simulink model "VCU_CS75_12_27_test"  (R2014a)
settings: Solver=FixedStepDiscrete  StartTime=0.0  StopTime=25  FixedStep=0.0005  RelTol=1e-3
undefined symbols (not defined in the file): D1, D2, D3, ecucoder_acal, ErrorSumMax1, ErrorSumMax2, ErrorSumMax3, I1, I2, I3, I_SW01_L, LaterlAngleCommand, LDW, P1, P2, P3, RemoteAcclPosition
libraries: simulink x913, ec5744lib x39
(part 11 of 30)

== system VCU_CS75_12_27_test/长安CS75底盘程序，20ms一次/Output/Subsystem/TransmitMessages10/LAS_29D ==
  LAS_LASWarningModeSelectionSts_in : Inport
  LAS_SLASwitchStatus_in : Inport  Port=2
  LAS_HMAEnableStatus_in : Inport  Port=3
  LAS_LASModeSelectionStatus_in : Inport  Port=4
  LAS_LdwSensitivityStatus_in : Inport  Port=5
  LAS_OverspeedSoundWarningEnSt_in : Inport  Port=6
  LAS_FatigueDectionEnableStatus_in : Inport  Port=7
  LAS_LDWShakeLevStatus_in : Inport  Port=8
  LAS_HostLaneLeftStatus_in : Inport  Port=9
  LAS_VoiceWarning_in : Inport  Port=10
  LAS_HostLaneRightStatus_in : Inport  Port=11
  LAS_OverspeedWarningEnableStatus_in : Inport  Port=12
  LAS_OverspeedSoundWarning_in : Inport  Port=13
  LAS_LLaneMarkerType_in : Inport  Port=14
  LAS_OverspeedVisualWarning_in : Inport  Port=15
  LAS_RLaneMarkerType_in : Inport  Port=16
  LAS_OverspeedWarningOffset_in : Inport  Port=17
  RollingConter_in : Inport  Port=18
  LAS_IACCEnableStatus_in : Inport  Port=19
  CRC_in : Inport  Port=20
  CRC : Subsystem
  Conv{1..8} (8 alike) : DataTypeConversion
  LAS_29D_DLC : Constant  Value=8  OutDataTypeStr=uint8
  LAS_29D_DLC_Out : Terminator
  LAS_29D_ID : Constant  Value=669  OutDataTypeStr=single
  LAS_29D_ID_Out : Terminator
  LAS_29D_mux : Mux  Inputs=8
  LAS_FatigueDectionEnableStatus : Subsystem
  LAS_HMAEnableStatus : Subsystem
  LAS_HostLaneLeftStatus : Subsystem
  LAS_HostLaneRightStatus : Subsystem
  LAS_IACCEnableStatus : Subsystem
  LAS_LASModeSelectionStatus : Subsystem
  LAS_LASWarningModeSelectionSts : Subsystem
  LAS_LDWShakeLevStatus : Subsystem
  LAS_LLaneMarkerType : Subsystem
  LAS_LdwSensitivityStatus : Subsystem
  LAS_OverspeedSoundWarning : Subsystem
  LAS_OverspeedSoundWarningEnSt : Subsystem
  LAS_OverspeedVisualWarning : Subsystem
  LAS_OverspeedWarningEnableStatus : Subsystem
  LAS_OverspeedWarningOffset : Subsystem
  LAS_RLaneMarkerType : Subsystem
  LAS_SLASwitchStatus : Subsystem
  LAS_VoiceWarning : Subsystem
  RollingConter : Subsystem
  or{1..8} (8 alike) : simulink/Logic and Bit Operations/Bitwise Operator  logicop=OR  UseBitMask=off  NumInputPorts=20  BitMask=bin2dec('11011001')  BitMaskRealWorld=Stored Integer
  output : Outport
  wires:
  LAS_29D_mux/1 -> output/1
  LAS_LASWarningModeSelectionSts/1(output1) -> or1/1
  LAS_LASWarningModeSelectionSts/2(output2) -> or2/1
  LAS_LASWarningModeSelectionSts/3(output3) -> or3/1
  LAS_LASWarningModeSelectionSts/4(output4) -> or4/1
  LAS_LASWarningModeSelectionSts/5(output5) -> or5/1
  LAS_LASWarningModeSelectionSts/6(output6) -> or6/1
  LAS_LASWarningModeSelectionSts/7(output7) -> or7/1
  LAS_LASWarningModeSelectionSts/8(output8) -> or8/1
  LAS_SLASwitchStatus/1(output1) -> or1/2
  LAS_SLASwitchStatus/2(output2) -> or2/2
  LAS_SLASwitchStatus/3(output3) -> or3/2
  LAS_SLASwitchStatus/4(output4) -> or4/2
  LAS_SLASwitchStatus/5(output5) -> or5/2
  LAS_SLASwitchStatus/6(output6) -> or6/2
  LAS_SLASwitchStatus/7(output7) -> or7/2
  LAS_SLASwitchStatus/8(output8) -> or8/2
  LAS_HMAEnableStatus/1(output1) -> or1/3
  LAS_HMAEnableStatus/2(output2) -> or2/3
  LAS_HMAEnableStatus/3(output3) -> or3/3
  LAS_HMAEnableStatus/4(output4) -> or4/3
  LAS_HMAEnableStatus/5(output5) -> or5/3
  LAS_HMAEnableStatus/6(output6) -> or6/3
  LAS_HMAEnableStatus/7(output7) -> or7/3
  LAS_HMAEnableStatus/8(output8) -> or8/3
  LAS_LASModeSelectionStatus/1(output1) -> or1/4
  LAS_LASModeSelectionStatus/2(output2) -> or2/4
  LAS_LASModeSelectionStatus/3(output3) -> or3/4
  LAS_LASModeSelectionStatus/4(output4) -> or4/4
  LAS_LASModeSelectionStatus/5(output5) -> or5/4
  LAS_LASModeSelectionStatus/6(output6) -> or6/4
  LAS_LASModeSelectionStatus/7(output7) -> or7/4
  LAS_LASModeSelectionStatus/8(output8) -> or8/4
  LAS_LdwSensitivityStatus/1(output1) -> or1/5
  LAS_LdwSensitivityStatus/2(output2) -> or2/5
  LAS_LdwSensitivityStatus/3(output3) -> or3/5
  LAS_LdwSensitivityStatus/4(output4) -> or4/5
  LAS_LdwSensitivityStatus/5(output5) -> or5/5
  LAS_LdwSensitivityStatus/6(output6) -> or6/5
  LAS_LdwSensitivityStatus/7(output7) -> or7/5
  LAS_LdwSensitivityStatus/8(output8) -> or8/5
  LAS_OverspeedSoundWarningEnSt/1(output1) -> or1/6
  LAS_OverspeedSoundWarningEnSt/2(output2) -> or2/6
  LAS_OverspeedSoundWarningEnSt/3(output3) -> or3/6
  LAS_OverspeedSoundWarningEnSt/4(output4) -> or4/6
  LAS_OverspeedSoundWarningEnSt/5(output5) -> or5/6
  LAS_OverspeedSoundWarningEnSt/6(output6) -> or6/6
  LAS_OverspeedSoundWarningEnSt/7(output7) -> or7/6
  LAS_OverspeedSoundWarningEnSt/8(output8) -> or8/6
  LAS_FatigueDectionEnableStatus/1(output1) -> or1/7
  LAS_FatigueDectionEnableStatus/2(output2) -> or2/7
  LAS_FatigueDectionEnableStatus/3(output3) -> or3/7
  LAS_FatigueDectionEnableStatus/4(output4) -> or4/7
  LAS_FatigueDectionEnableStatus/5(output5) -> or5/7
  LAS_FatigueDectionEnableStatus/6(output6) -> or6/7
  LAS_FatigueDectionEnableStatus/7(output7) -> or7/7
  LAS_FatigueDectionEnableStatus/8(output8) -> or8/7
  LAS_LDWShakeLevStatus/1(output1) -> or1/8
  LAS_LDWShakeLevStatus/2(output2) -> or2/8
  LAS_LDWShakeLevStatus/3(output3) -> or3/8
  LAS_LDWShakeLevStatus/4(output4) -> or4/8
  LAS_LDWShakeLevStatus/5(output5) -> or5/8
  LAS_LDWShakeLevStatus/6(output6) -> or6/8
  LAS_LDWShakeLevStatus/7(output7) -> or7/8
  LAS_LDWShakeLevStatus/8(output8) -> or8/8
  LAS_HostLaneLeftStatus/1(output1) -> or1/9
  LAS_HostLaneLeftStatus/2(output2) -> or2/9
  LAS_HostLaneLeftStatus/3(output3) -> or3/9
  LAS_HostLaneLeftStatus/4(output4) -> or4/9
  LAS_HostLaneLeftStatus/5(output5) -> or5/9
  LAS_HostLaneLeftStatus/6(output6) -> or6/9
  LAS_HostLaneLeftStatus/7(output7) -> or7/9
  LAS_HostLaneLeftStatus/8(output8) -> or8/9
  LAS_VoiceWarning/1(output1) -> or1/10
  LAS_VoiceWarning/2(output2) -> or2/10
  LAS_VoiceWarning/3(output3) -> or3/10
  LAS_VoiceWarning/4(output4) -> or4/10
  LAS_VoiceWarning/5(output5) -> or5/10
  LAS_VoiceWarning/6(output6) -> or6/10
  LAS_VoiceWarning/7(output7) -> or7/10
  LAS_VoiceWarning/8(output8) -> or8/10
  LAS_HostLaneRightStatus/1(output1) -> or1/11
  LAS_HostLaneRightStatus/2(output2) -> or2/11
  LAS_HostLaneRightStatus/3(output3) -> or3/11
  LAS_HostLaneRightStatus/4(output4) -> or4/11
  LAS_HostLaneRightStatus/5(output5) -> or5/11
  LAS_HostLaneRightStatus/6(output6) -> or6/11
  LAS_HostLaneRightStatus/7(output7) -> or7/11
  LAS_HostLaneRightStatus/8(output8) -> or8/11
  LAS_OverspeedWarningEnableStatus/1(output1) -> or1/12
  LAS_OverspeedWarningEnableStatus/2(output2) -> or2/12
  LAS_OverspeedWarningEnableStatus/3(output3) -> or3/12
  LAS_OverspeedWarningEnableStatus/4(output4) -> or4/12
  LAS_OverspeedWarningEnableStatus/5(output5) -> or5/12
  LAS_OverspeedWarningEnableStatus/6(output6) -> or6/12
  LAS_OverspeedWarningEnableStatus/7(output7) -> or7/12
  LAS_OverspeedWarningEnableStatus/8(output8) -> or8/12
  LAS_OverspeedSoundWarning/1(output1) -> or1/13
  LAS_OverspeedSoundWarning/2(output2) -> or2/13
  LAS_OverspeedSoundWarning/3(output3) -> or3/13
  LAS_OverspeedSoundWarning/4(output4) -> or4/13
  LAS_OverspeedSoundWarning/5(output5) -> or5/13
  LAS_OverspeedSoundWarning/6(output6) -> or6/13
  LAS_OverspeedSoundWarning/7(output7) -> or7/13
  LAS_OverspeedSoundWarning/8(output8) -> or8/13
  LAS_LLaneMarkerType/1(output1) -> or1/14
  LAS_LLaneMarkerType/2(output2) -> or2/14
  LAS_LLaneMarkerType/3(output3) -> or3/14
  LAS_LLaneMarkerType/4(output4) -> or4/14
  LAS_LLaneMarkerType/5(output5) -> or5/14
  LAS_LLaneMarkerType/6(output6) -> or6/14
  LAS_LLaneMarkerType/7(output7) -> or7/14
  LAS_LLaneMarkerType/8(output8) -> or8/14
  LAS_OverspeedVisualWarning/1(output1) -> or1/15
  LAS_OverspeedVisualWarning/2(output2) -> or2/15
  LAS_OverspeedVisualWarning/3(output3) -> or3/15
  LAS_OverspeedVisualWarning/4(output4) -> or4/15
  LAS_OverspeedVisualWarning/5(output5) -> or5/15
  LAS_OverspeedVisualWarning/6(output6) -> or6/15
  LAS_OverspeedVisualWarning/7(output7) -> or7/15
  LAS_OverspeedVisualWarning/8(output8) -> or8/15
  LAS_RLaneMarkerType/1(output1) -> or1/16
  LAS_RLaneMarkerType/2(output2) -> or2/16
  LAS_RLaneMarkerType/3(output3) -> or3/16
  LAS_RLaneMarkerType/4(output4) -> or4/16
  LAS_RLaneMarkerType/5(output5) -> or5/16
  LAS_RLaneMarkerType/6(output6) -> or6/16
  LAS_RLaneMarkerType/7(output7) -> or7/16
  LAS_RLaneMarkerType/8(output8) -> or8/16
  LAS_OverspeedWarningOffset/1(output1) -> or1/17
  LAS_OverspeedWarningOffset/2(output2) -> or2/17
  LAS_OverspeedWarningOffset/3(output3) -> or3/17
  LAS_OverspeedWarningOffset/4(output4) -> or4/17
  LAS_OverspeedWarningOffset/5(output5) -> or5/17
  LAS_OverspeedWarningOffset/6(output6) -> or6/17
  LAS_OverspeedWarningOffset/7(output7) -> or7/17
  LAS_OverspeedWarningOffset/8(output8) -> or8/17
  RollingConter/1(output1) -> or1/18
  RollingConter/2(output2) -> or2/18
  RollingConter/3(output3) -> or3/18
  RollingConter/4(output4) -> or4/18
  RollingConter/5(output5) -> or5/18
  RollingConter/6(output6) -> or6/18
  RollingConter/7(output7) -> or7/18
  RollingConter/8(output8) -> or8/18
  LAS_IACCEnableStatus/1(output1) -> or1/19
  LAS_IACCEnableStatus/2(output2) -> or2/19
  LAS_IACCEnableStatus/3(output3) -> or3/19
  LAS_IACCEnableStatus/4(output4) -> or4/19
  LAS_IACCEnableStatus/5(output5) -> or5/19
  LAS_IACCEnableStatus/6(output6) -> or6/19
  LAS_IACCEnableStatus/7(output7) -> or7/19
  LAS_IACCEnableStatus/8(output8) -> or8/19
  CRC/1(output1) -> or1/20
  CRC/2(output2) -> or2/20
  CRC/3(output3) -> or3/20
  CRC/4(output4) -> or4/20
  CRC/5(output5) -> or5/20
  CRC/6(output6) -> or6/20
  CRC/7(output7) -> or7/20
  CRC/8(output8) -> or8/20
  or1/1 -> Conv1/1
  Conv1/1 -> LAS_29D_mux/1
  or2/1 -> Conv2/1
  Conv2/1 -> LAS_29D_mux/2
  or3/1 -> Conv3/1
  Conv3/1 -> LAS_29D_mux/3
  or4/1 -> Conv4/1
  Conv4/1 -> LAS_29D_mux/4
  or5/1 -> Conv5/1
  Conv5/1 -> LAS_29D_mux/5
  or6/1 -> Conv6/1
  Conv6/1 -> LAS_29D_mux/6
  or7/1 -> Conv7/1
  Conv7/1 -> LAS_29D_mux/7
  or8/1 -> Conv8/1
  Conv8/1 -> LAS_29D_mux/8
  LAS_29D_ID/1 -> LAS_29D_ID_Out/1
  LAS_29D_DLC/1 -> LAS_29D_DLC_Out/1
  LAS_LASWarningModeSelectionSts_in/1 -> LAS_LASWarningModeSelectionSts/1(LAS_LASWarningModeSelectionSts)
  LAS_SLASwitchStatus_in/1 -> LAS_SLASwitchStatus/1(LAS_SLASwitchStatus)
  LAS_HMAEnableStatus_in/1 -> LAS_HMAEnableStatus/1(LAS_HMAEnableStatus)
  LAS_LASModeSelectionStatus_in/1 -> LAS_LASModeSelectionStatus/1(LAS_LASModeSelectionStatus)
  LAS_LdwSensitivityStatus_in/1 -> LAS_LdwSensitivityStatus/1(LAS_LdwSensitivityStatus)
  LAS_OverspeedSoundWarningEnSt_in/1 -> LAS_OverspeedSoundWarningEnSt/1(LAS_OverspeedSoundWarningEnSt)
  LAS_FatigueDectionEnableStatus_in/1 -> LAS_FatigueDectionEnableStatus/1(LAS_FatigueDectionEnableStatus)
  LAS_LDWShakeLevStatus_in/1 -> LAS_LDWShakeLevStatus/1(LAS_LDWShakeLevStatus)
  LAS_HostLaneLeftStatus_in/1 -> LAS_HostLaneLeftStatus/1(LAS_HostLaneLeftStatus)
  LAS_VoiceWarning_in/1 -> LAS_VoiceWarning/1(LAS_VoiceWarning)
  LAS_HostLaneRightStatus_in/1 -> LAS_HostLaneRightStatus/1(LAS_HostLaneRightStatus)
  LAS_OverspeedWarningEnableStatus_in/1 -> LAS_OverspeedWarningEnableStatus/1(LAS_OverspeedWarningEnableStatus)
  LAS_OverspeedSoundWarning_in/1 -> LAS_OverspeedSoundWarning/1(LAS_OverspeedSoundWarning)
  LAS_LLaneMarkerType_in/1 -> LAS_LLaneMarkerType/1(LAS_LLaneMarkerType)
  LAS_OverspeedVisualWarning_in/1 -> LAS_OverspeedVisualWarning/1(LAS_OverspeedVisualWarning)
  LAS_RLaneMarkerType_in/1 -> LAS_RLaneMarkerType/1(LAS_RLaneMarkerType)
  LAS_OverspeedWarningOffset_in/1 -> LAS_OverspeedWarningOffset/1(LAS_OverspeedWarningOffset)
  RollingConter_in/1 -> RollingConter/1(RollingConter)
  LAS_IACCEnableStatus_in/1 -> LAS_IACCEnableStatus/1(LAS_IACCEnableStatus)
  CRC_in/1 -> CRC/1(CRC)

== system VCU_CS75_12_27_test/长安CS75底盘程序，20ms一次/Output/Subsystem/TransmitMessages11/GW_LCDAL_2EA ==
  LCDAL_SystemStatus_in : Inport
  LCDAL_BSDLCAEnableStatus_in : Inport  Port=2
  LCDAL_BSDLCAAlert_in : Inport  Port=3
  LCDAL_BSDLCAStatus_in : Inport  Port=4
  LCDAL_CTAEnableStatus_in : Inport  Port=5
  LCDAL_CTAAlert_in : Inport  Port=6
  LCDAL_CTAStatus_in : Inport  Port=7
  LCDAL_RCWEnableStatus_in : Inport  Port=8
  LCDAL_RCWAlert_in : Inport  Port=9
  LCDAL_RCWStatus_in : Inport  Port=10
  LCDAL_RCWSoundEnableStatus_in : Inport  Port=11
  LCDAL_SEAEnableStatus_in : Inport  Port=12
  LCDAL_SEAAlert_in : Inport  Port=13
  LCDAL_SEAStatus_in : Inport  Port=14
  LCDAL_AudioWarningEnableStatus_in : Inport  Port=15
  LCDAL_LockCtrlEnableStatus_in : Inport  Port=16
  LCDAL_LCATTCSettingStatus_in : Inport  Port=17
  Conv{1..8} (8 alike) : DataTypeConversion
  GW_LCDAL_2EA_DLC : Constant  Value=8  OutDataTypeStr=uint8
  GW_LCDAL_2EA_DLC_Out : Terminator
  GW_LCDAL_2EA_ID : Constant  Value=746  OutDataTypeStr=single
  GW_LCDAL_2EA_ID_Out : Terminator
  GW_LCDAL_2EA_mux : Mux  Inputs=8
  LCDAL_AudioWarningEnableStatus : Subsystem
  LCDAL_BSDLCAAlert : Subsystem
  LCDAL_BSDLCAEnableStatus : Subsystem
  LCDAL_BSDLCAStatus : Subsystem
  LCDAL_CTAAlert : Subsystem
  LCDAL_CTAEnableStatus : Subsystem
  LCDAL_CTAStatus : Subsystem
  LCDAL_LCATTCSettingStatus : Subsystem
  LCDAL_LockCtrlEnableStatus : Subsystem
  LCDAL_RCWAlert : Subsystem
  LCDAL_RCWEnableStatus : Subsystem
  LCDAL_RCWSoundEnableStatus : Subsystem
  LCDAL_RCWStatus : Subsystem
  LCDAL_SEAAlert : Subsystem
  LCDAL_SEAEnableStatus : Subsystem
  LCDAL_SEAStatus : Subsystem
  LCDAL_SystemStatus : Subsystem
  or{1..8} (8 alike) : simulink/Logic and Bit Operations/Bitwise Operator  logicop=OR  UseBitMask=off  NumInputPorts=17  BitMask=bin2dec('11011001')  BitMaskRealWorld=Stored Integer
  output : Outport
  wires:
  LCDAL_LCATTCSettingStatus_in/1 -> LCDAL_LCATTCSettingStatus/1(LCDAL_LCATTCSettingStatus)
  LCDAL_LockCtrlEnableStatus_in/1 -> LCDAL_LockCtrlEnableStatus/1(LCDAL_LockCtrlEnableStatus)
  LCDAL_AudioWarningEnableStatus_in/1 -> LCDAL_AudioWarningEnableStatus/1(LCDAL_AudioWarningEnableStatus)
  LCDAL_SEAStatus_in/1 -> LCDAL_SEAStatus/1(LCDAL_SEAStatus)
  LCDAL_SEAAlert_in/1 -> LCDAL_SEAAlert/1(LCDAL_SEAAlert)
  LCDAL_SEAEnableStatus_in/1 -> LCDAL_SEAEnableStatus/1(LCDAL_SEAEnableStatus)
  LCDAL_RCWSoundEnableStatus_in/1 -> LCDAL_RCWSoundEnableStatus/1(LCDAL_RCWSoundEnableStatus)
  LCDAL_RCWStatus_in/1 -> LCDAL_RCWStatus/1(LCDAL_RCWStatus)
  LCDAL_RCWAlert_in/1 -> LCDAL_RCWAlert/1(LCDAL_RCWAlert)
  LCDAL_RCWEnableStatus_in/1 -> LCDAL_RCWEnableStatus/1(LCDAL_RCWEnableStatus)
  LCDAL_CTAStatus_in/1 -> LCDAL_CTAStatus/1(LCDAL_CTAStatus)
  LCDAL_CTAAlert_in/1 -> LCDAL_CTAAlert/1(LCDAL_CTAAlert)
  LCDAL_CTAEnableStatus_in/1 -> LCDAL_CTAEnableStatus/1(LCDAL_CTAEnableStatus)
  LCDAL_BSDLCAStatus_in/1 -> LCDAL_BSDLCAStatus/1(LCDAL_BSDLCAStatus)
  LCDAL_BSDLCAAlert_in/1 -> LCDAL_BSDLCAAlert/1(LCDAL_BSDLCAAlert)
  LCDAL_BSDLCAEnableStatus_in/1 -> LCDAL_BSDLCAEnableStatus/1(LCDAL_BSDLCAEnableStatus)
  LCDAL_SystemStatus_in/1 -> LCDAL_SystemStatus/1(LCDAL_SystemStatus)
  GW_LCDAL_2EA_DLC/1 -> GW_LCDAL_2EA_DLC_Out/1
  GW_LCDAL_2EA_ID/1 -> GW_LCDAL_2EA_ID_Out/1
  Conv8/1 -> GW_LCDAL_2EA_mux/8
  or8/1 -> Conv8/1
  Conv7/1 -> GW_LCDAL_2EA_mux/7
  or7/1 -> Conv7/1
  Conv6/1 -> GW_LCDAL_2EA_mux/6
  or6/1 -> Conv6/1
  Conv5/1 -> GW_LCDAL_2EA_mux/5
  or5/1 -> Conv5/1
  Conv4/1 -> GW_LCDAL_2EA_mux/4
  or4/1 -> Conv4/1
  Conv3/1 -> GW_LCDAL_2EA_mux/3
  or3/1 -> Conv3/1
  Conv2/1 -> GW_LCDAL_2EA_mux/2
  or2/1 -> Conv2/1
  Conv1/1 -> GW_LCDAL_2EA_mux/1
  or1/1 -> Conv1/1
  LCDAL_LCATTCSettingStatus/8(output8) -> or8/17
  LCDAL_LCATTCSettingStatus/7(output7) -> or7/17
  LCDAL_LCATTCSettingStatus/6(output6) -> or6/17
  LCDAL_LCATTCSettingStatus/5(output5) -> or5/17
  LCDAL_LCATTCSettingStatus/4(output4) -> or4/17
  LCDAL_LCATTCSettingStatus/3(output3) -> or3/17
  LCDAL_LCATTCSettingStatus/2(output2) -> or2/17
  LCDAL_LCATTCSettingStatus/1(output1) -> or1/17
  LCDAL_LockCtrlEnableStatus/8(output8) -> or8/16
  LCDAL_LockCtrlEnableStatus/7(output7) -> or7/16
  LCDAL_LockCtrlEnableStatus/6(output6) -> or6/16
  LCDAL_LockCtrlEnableStatus/5(output5) -> or5/16
  LCDAL_LockCtrlEnableStatus/4(output4) -> or4/16
  LCDAL_LockCtrlEnableStatus/3(output3) -> or3/16
  LCDAL_LockCtrlEnableStatus/2(output2) -> or2/16
  LCDAL_LockCtrlEnableStatus/1(output1) -> or1/16
  LCDAL_AudioWarningEnableStatus/8(output8) -> or8/15
  LCDAL_AudioWarningEnableStatus/7(output7) -> or7/15
  LCDAL_AudioWarningEnableStatus/6(output6) -> or6/15
  LCDAL_AudioWarningEnableStatus/5(output5) -> or5/15
  LCDAL_AudioWarningEnableStatus/4(output4) -> or4/15
  LCDAL_AudioWarningEnableStatus/3(output3) -> or3/15
  LCDAL_AudioWarningEnableStatus/2(output2) -> or2/15
  LCDAL_AudioWarningEnableStatus/1(output1) -> or1/15
  LCDAL_SEAStatus/8(output8) -> or8/14
  LCDAL_SEAStatus/7(output7) -> or7/14
  LCDAL_SEAStatus/6(output6) -> or6/14
  LCDAL_SEAStatus/5(output5) -> or5/14
  LCDAL_SEAStatus/4(output4) -> or4/14
  LCDAL_SEAStatus/3(output3) -> or3/14
  LCDAL_SEAStatus/2(output2) -> or2/14
  LCDAL_SEAStatus/1(output1) -> or1/14
  LCDAL_SEAAlert/8(output8) -> or8/13
  LCDAL_SEAAlert/7(output7) -> or7/13
  LCDAL_SEAAlert/6(output6) -> or6/13
  LCDAL_SEAAlert/5(output5) -> or5/13
  LCDAL_SEAAlert/4(output4) -> or4/13
  LCDAL_SEAAlert/3(output3) -> or3/13
  LCDAL_SEAAlert/2(output2) -> or2/13
  LCDAL_SEAAlert/1(output1) -> or1/13
  LCDAL_SEAEnableStatus/8(output8) -> or8/12
  LCDAL_SEAEnableStatus/7(output7) -> or7/12
  LCDAL_SEAEnableStatus/6(output6) -> or6/12
  LCDAL_SEAEnableStatus/5(output5) -> or5/12
  LCDAL_SEAEnableStatus/4(output4) -> or4/12
  LCDAL_SEAEnableStatus/3(output3) -> or3/12
  LCDAL_SEAEnableStatus/2(output2) -> or2/12
  LCDAL_SEAEnableStatus/1(output1) -> or1/12
  LCDAL_RCWSoundEnableStatus/8(output8) -> or8/11
  LCDAL_RCWSoundEnableStatus/7(output7) -> or7/11
  LCDAL_RCWSoundEnableStatus/6(output6) -> or6/11
  LCDAL_RCWSoundEnableStatus/5(output5) -> or5/11
  LCDAL_RCWSoundEnableStatus/4(output4) -> or4/11
  LCDAL_RCWSoundEnableStatus/3(output3) -> or3/11
  LCDAL_RCWSoundEnableStatus/2(output2) -> or2/11
  LCDAL_RCWSoundEnableStatus/1(output1) -> or1/11
  LCDAL_RCWStatus/8(output8) -> or8/10
  LCDAL_RCWStatus/7(output7) -> or7/10
  LCDAL_RCWStatus/6(output6) -> or6/10
  LCDAL_RCWStatus/5(output5) -> or5/10
  LCDAL_RCWStatus/4(output4) -> or4/10
  LCDAL_RCWStatus/3(output3) -> or3/10
  LCDAL_RCWStatus/2(output2) -> or2/10
  LCDAL_RCWStatus/1(output1) -> or1/10
  LCDAL_RCWAlert/8(output8) -> or8/9
  LCDAL_RCWAlert/7(output7) -> or7/9
  LCDAL_RCWAlert/6(output6) -> or6/9
  LCDAL_RCWAlert/5(output5) -> or5/9
  LCDAL_RCWAlert/4(output4) -> or4/9
  LCDAL_RCWAlert/3(output3) -> or3/9
  LCDAL_RCWAlert/2(output2) -> or2/9
  LCDAL_RCWAlert/1(output1) -> or1/9
  LCDAL_RCWEnableStatus/8(output8) -> or8/8
  LCDAL_RCWEnableStatus/7(output7) -> or7/8
  LCDAL_RCWEnableStatus/6(output6) -> or6/8
  LCDAL_RCWEnableStatus/5(output5) -> or5/8
  LCDAL_RCWEnableStatus/4(output4) -> or4/8
  LCDAL_RCWEnableStatus/3(output3) -> or3/8
  LCDAL_RCWEnableStatus/2(output2) -> or2/8
  LCDAL_RCWEnableStatus/1(output1) -> or1/8
  LCDAL_CTAStatus/8(output8) -> or8/7
  LCDAL_CTAStatus/7(output7) -> or7/7
  LCDAL_CTAStatus/6(output6) -> or6/7
  LCDAL_CTAStatus/5(output5) -> or5/7
  LCDAL_CTAStatus/4(output4) -> or4/7
  LCDAL_CTAStatus/3(output3) -> or3/7
  LCDAL_CTAStatus/2(output2) -> or2/7
  LCDAL_CTAStatus/1(output1) -> or1/7
  LCDAL_CTAAlert/8(output8) -> or8/6
  LCDAL_CTAAlert/7(output7) -> or7/6
  LCDAL_CTAAlert/6(output6) -> or6/6
  LCDAL_CTAAlert/5(output5) -> or5/6
  LCDAL_CTAAlert/4(output4) -> or4/6
  LCDAL_CTAAlert/3(output3) -> or3/6
  LCDAL_CTAAlert/2(output2) -> or2/6
  LCDAL_CTAAlert/1(output1) -> or1/6
  LCDAL_CTAEnableStatus/8(output8) -> or8/5
  LCDAL_CTAEnableStatus/7(output7) -> or7/5
  LCDAL_CTAEnableStatus/6(output6) -> or6/5
  LCDAL_CTAEnableStatus/5(output5) -> or5/5
  LCDAL_CTAEnableStatus/4(output4) -> or4/5
  LCDAL_CTAEnableStatus/3(output3) -> or3/5
  LCDAL_CTAEnableStatus/2(output2) -> or2/5
  LCDAL_CTAEnableStatus/1(output1) -> or1/5
  LCDAL_BSDLCAStatus/8(output8) -> or8/4
  LCDAL_BSDLCAStatus/7(output7) -> or7/4
  LCDAL_BSDLCAStatus/6(output6) -> or6/4
  LCDAL_BSDLCAStatus/5(output5) -> or5/4
  LCDAL_BSDLCAStatus/4(output4) -> or4/4
  LCDAL_BSDLCAStatus/3(output3) -> or3/4
  LCDAL_BSDLCAStatus/2(output2) -> or2/4
  LCDAL_BSDLCAStatus/1(output1) -> or1/4
  LCDAL_BSDLCAAlert/8(output8) -> or8/3
  LCDAL_BSDLCAAlert/7(output7) -> or7/3
  LCDAL_BSDLCAAlert/6(output6) -> or6/3
  LCDAL_BSDLCAAlert/5(output5) -> or5/3
  LCDAL_BSDLCAAlert/4(output4) -> or4/3
  LCDAL_BSDLCAAlert/3(output3) -> or3/3
  LCDAL_BSDLCAAlert/2(output2) -> or2/3
  LCDAL_BSDLCAAlert/1(output1) -> or1/3
  LCDAL_BSDLCAEnableStatus/8(output8) -> or8/2
  LCDAL_BSDLCAEnableStatus/7(output7) -> or7/2
  LCDAL_BSDLCAEnableStatus/6(output6) -> or6/2
  LCDAL_BSDLCAEnableStatus/5(output5) -> or5/2
  LCDAL_BSDLCAEnableStatus/4(output4) -> or4/2
  LCDAL_BSDLCAEnableStatus/3(output3) -> or3/2
  LCDAL_BSDLCAEnableStatus/2(output2) -> or2/2
  LCDAL_BSDLCAEnableStatus/1(output1) -> or1/2
  LCDAL_SystemStatus/8(output8) -> or8/1
  LCDAL_SystemStatus/7(output7) -> or7/1
  LCDAL_SystemStatus/6(output6) -> or6/1
  LCDAL_SystemStatus/5(output5) -> or5/1
  LCDAL_SystemStatus/4(output4) -> or4/1
  LCDAL_SystemStatus/3(output3) -> or3/1
  LCDAL_SystemStatus/2(output2) -> or2/1
  LCDAL_SystemStatus/1(output1) -> or1/1
  GW_LCDAL_2EA_mux/1 -> output/1

== system VCU_CS75_12_27_test/长安CS75底盘程序，20ms一次/Output/Subsystem/TransmitMessages13/GW_LCDAR_2FA ==
  LCDAR_SystemStatus_in : Inport
  LCDAR_BSDLCAAlert_in : Inport  Port=2
  LCDAR_BSDLCAStatus_in : Inport  Port=3
  LCDAR_CTAAlert_in : Inport  Port=4
  LCDAR_CTAStatus_in : Inport  Port=5
  LCDAR_RCWAlert_in : Inport  Port=6
  LCDAR_RCWStatus_in : Inport  Port=7
  LCDAR_SEAAlert_in : Inport  Port=8
  LCDAR_SEAStatus_in : Inport  Port=9
  Conv{1..8} (8 alike) : DataTypeConversion
  GW_LCDAR_2FA_DLC : Constant  Value=8  OutDataTypeStr=uint8
  GW_LCDAR_2FA_DLC_Out : Terminator
  GW_LCDAR_2FA_ID : Constant  Value=762  OutDataTypeStr=single
  GW_LCDAR_2FA_ID_Out : Terminator
  GW_LCDAR_2FA_mux : Mux  Inputs=8
  LCDAR_BSDLCAAlert : Subsystem
  LCDAR_BSDLCAStatus : Subsystem
  LCDAR_CTAAlert : Subsystem
  LCDAR_CTAStatus : Subsystem
  LCDAR_RCWAlert : Subsystem
  LCDAR_RCWStatus : Subsystem
  LCDAR_SEAAlert : Subsystem
  LCDAR_SEAStatus : Subsystem
  LCDAR_SystemStatus : Subsystem
  or{1..8} (8 alike) : simulink/Logic and Bit Operations/Bitwise Operator  logicop=OR  UseBitMask=off  NumInputPorts=9  BitMask=bin2dec('11011001')  BitMaskRealWorld=Stored Integer
  output : Outport
  wires:
  GW_LCDAR_2FA_mux/1 -> output/1
  LCDAR_SystemStatus/1(output1) -> or1/1
  LCDAR_SystemStatus/2(output2) -> or2/1
  LCDAR_SystemStatus/3(output3) -> or3/1
  LCDAR_SystemStatus/4(output4) -> or4/1
  LCDAR_SystemStatus/5(output5) -> or5/1
  LCDAR_SystemStatus/6(output6) -> or6/1
  LCDAR_SystemStatus/7(output7) -> or7/1
  LCDAR_SystemStatus/8(output8) -> or8/1
  LCDAR_BSDLCAAlert/1(output1) -> or1/2
  LCDAR_BSDLCAAlert/2(output2) -> or2/2
  LCDAR_BSDLCAAlert/3(output3) -> or3/2
  LCDAR_BSDLCAAlert/4(output4) -> or4/2
  LCDAR_BSDLCAAlert/5(output5) -> or5/2
  LCDAR_BSDLCAAlert/6(output6) -> or6/2
  LCDAR_BSDLCAAlert/7(output7) -> or7/2
  LCDAR_BSDLCAAlert/8(output8) -> or8/2
  LCDAR_BSDLCAStatus/1(output1) -> or1/3
  LCDAR_BSDLCAStatus/2(output2) -> or2/3
  LCDAR_BSDLCAStatus/3(output3) -> or3/3
  LCDAR_BSDLCAStatus/4(output4) -> or4/3
  LCDAR_BSDLCAStatus/5(output5) -> or5/3
  LCDAR_BSDLCAStatus/6(output6) -> or6/3
  LCDAR_BSDLCAStatus/7(output7) -> or7/3
  LCDAR_BSDLCAStatus/8(output8) -> or8/3
  LCDAR_CTAAlert/1(output1) -> or1/4
  LCDAR_CTAAlert/2(output2) -> or2/4
  LCDAR_CTAAlert/3(output3) -> or3/4
  LCDAR_CTAAlert/4(output4) -> or4/4
  LCDAR_CTAAlert/5(output5) -> or5/4
  LCDAR_CTAAlert/6(output6) -> or6/4
  LCDAR_CTAAlert/7(output7) -> or7/4
  LCDAR_CTAAlert/8(output8) -> or8/4
  LCDAR_CTAStatus/1(output1) -> or1/5
  LCDAR_CTAStatus/2(output2) -> or2/5
  LCDAR_CTAStatus/3(output3) -> or3/5
  LCDAR_CTAStatus/4(output4) -> or4/5
  LCDAR_CTAStatus/5(output5) -> or5/5
  LCDAR_CTAStatus/6(output6) -> or6/5
  LCDAR_CTAStatus/7(output7) -> or7/5
  LCDAR_CTAStatus/8(output8) -> or8/5
  LCDAR_RCWAlert/1(output1) -> or1/6
  LCDAR_RCWAlert/2(output2) -> or2/6
  LCDAR_RCWAlert/3(output3) -> or3/6
  LCDAR_RCWAlert/4(output4) -> or4/6
  LCDAR_RCWAlert/5(output5) -> or5/6
  LCDAR_RCWAlert/6(output6) -> or6/6
  LCDAR_RCWAlert/7(output7) -> or7/6
  LCDAR_RCWAlert/8(output8) -> or8/6
  LCDAR_RCWStatus/1(output1) -> or1/7
  LCDAR_RCWStatus/2(output2) -> or2/7
  LCDAR_RCWStatus/3(output3) -> or3/7
  LCDAR_RCWStatus/4(output4) -> or4/7
  LCDAR_RCWStatus/5(output5) -> or5/7
  LCDAR_RCWStatus/6(output6) -> or6/7
  LCDAR_RCWStatus/7(output7) -> or7/7
  LCDAR_RCWStatus/8(output8) -> or8/7
  LCDAR_SEAAlert/1(output1) -> or1/8
  LCDAR_SEAAlert/2(output2) -> or2/8
  LCDAR_SEAAlert/3(output3) -> or3/8
  LCDAR_SEAAlert/4(output4) -> or4/8
  LCDAR_SEAAlert/5(output5) -> or5/8
  LCDAR_SEAAlert/6(output6) -> or6/8
  LCDAR_SEAAlert/7(output7) -> or7/8
  LCDAR_SEAAlert/8(output8) -> or8/8
  LCDAR_SEAStatus/1(output1) -> or1/9
  LCDAR_SEAStatus/2(output2) -> or2/9
  LCDAR_SEAStatus/3(output3) -> or3/9
  LCDAR_SEAStatus/4(output4) -> or4/9
  LCDAR_SEAStatus/5(output5) -> or5/9
  LCDAR_SEAStatus/6(output6) -> or6/9
  LCDAR_SEAStatus/7(output7) -> or7/9
  LCDAR_SEAStatus/8(output8) -> or8/9
  or1/1 -> Conv1/1
  Conv1/1 -> GW_LCDAR_2FA_mux/1
  or2/1 -> Conv2/1
  Conv2/1 -> GW_LCDAR_2FA_mux/2
  or3/1 -> Conv3/1
  Conv3/1 -> GW_LCDAR_2FA_mux/3
  or4/1 -> Conv4/1
  Conv4/1 -> GW_LCDAR_2FA_mux/4
  or5/1 -> Conv5/1
  Conv5/1 -> GW_LCDAR_2FA_mux/5
  or6/1 -> Conv6/1
  Conv6/1 -> GW_LCDAR_2FA_mux/6
  or7/1 -> Conv7/1
  Conv7/1 -> GW_LCDAR_2FA_mux/7
  or8/1 -> Conv8/1
  Conv8/1 -> GW_LCDAR_2FA_mux/8
  GW_LCDAR_2FA_ID/1 -> GW_LCDAR_2FA_ID_Out/1
  GW_LCDAR_2FA_DLC/1 -> GW_LCDAR_2FA_DLC_Out/1
  LCDAR_SystemStatus_in/1 -> LCDAR_SystemStatus/1(LCDAR_SystemStatus)
  LCDAR_BSDLCAAlert_in/1 -> LCDAR_BSDLCAAlert/1(LCDAR_BSDLCAAlert)
  LCDAR_BSDLCAStatus_in/1 -> LCDAR_BSDLCAStatus/1(LCDAR_BSDLCAStatus)
  LCDAR_CTAAlert_in/1 -> LCDAR_CTAAlert/1(LCDAR_CTAAlert)
  LCDAR_CTAStatus_in/1 -> LCDAR_CTAStatus/1(LCDAR_CTAStatus)
  LCDAR_RCWAlert_in/1 -> LCDAR_RCWAlert/1(LCDAR_RCWAlert)
  LCDAR_RCWStatus_in/1 -> LCDAR_RCWStatus/1(LCDAR_RCWStatus)
  LCDAR_SEAAlert_in/1 -> LCDAR_SEAAlert/1(LCDAR_SEAAlert)
  LCDAR_SEAStatus_in/1 -> LCDAR_SEAStatus/1(LCDAR_SEAStatus)

== system VCU_CS75_12_27_test/长安CS75底盘程序，20ms一次/Output/Subsystem/TransmitMessages14/LAS_2AD ==
  LAS_TargetBasedLateralCOntrol_in : Inport
  LAS_DriverHandsOff_in : Inport  Port=2
  LAS_IACCMode_in : Inport  Port=3
  LAS_IACCTextInfoForDriver_in : Inport  Port=4
  RollingConter_in : Inport  Port=5
  CRC_in : Inport  Port=6
  CRC : Subsystem
  Conv{1..8} (8 alike) : DataTypeConversion
  LAS_2AD_DLC : Constant  Value=8  OutDataTypeStr=uint8
  LAS_2AD_DLC_Out : Terminator
  LAS_2AD_ID : Constant  Value=685  OutDataTypeStr=single
  LAS_2AD_ID_Out : Terminator
  LAS_2AD_mux : Mux  Inputs=8
  LAS_DriverHandsOff : Subsystem
  LAS_IACCMode : Subsystem
  LAS_IACCTextInfoForDriver : Subsystem
  LAS_TargetBasedLateralCOntrol : Subsystem
  RollingConter : Subsystem
  or{1..8} (8 alike) : simulink/Logic and Bit Operations/Bitwise Operator  logicop=OR  UseBitMask=off  NumInputPorts=6  BitMask=bin2dec('11011001')  BitMaskRealWorld=Stored Integer
  output : Outport
  wires:
  CRC_in/1 -> CRC/1(CRC)
  RollingConter_in/1 -> RollingConter/1(RollingConter)
  LAS_IACCTextInfoForDriver_in/1 -> LAS_IACCTextInfoForDriver/1(LAS_IACCTextInfoForDriver)
  LAS_IACCMode_in/1 -> LAS_IACCMode/1(LAS_IACCMode)
  LAS_DriverHandsOff_in/1 -> LAS_DriverHandsOff/1(LAS_DriverHandsOff)
  LAS_TargetBasedLateralCOntrol_in/1 -> LAS_TargetBasedLateralCOntrol/1(LAS_TargetBasedLateralCOntrol)
  LAS_2AD_DLC/1 -> LAS_2AD_DLC_Out/1
  LAS_2AD_ID/1 -> LAS_2AD_ID_Out/1
  Conv8/1 -> LAS_2AD_mux/8
  or8/1 -> Conv8/1
  Conv7/1 -> LAS_2AD_mux/7
  or7/1 -> Conv7/1
  Conv6/1 -> LAS_2AD_mux/6
  or6/1 -> Conv6/1
  Conv5/1 -> LAS_2AD_mux/5
  or5/1 -> Conv5/1
  Conv4/1 -> LAS_2AD_mux/4
  or4/1 -> Conv4/1
  Conv3/1 -> LAS_2AD_mux/3
  or3/1 -> Conv3/1
  Conv2/1 -> LAS_2AD_mux/2
  or2/1 -> Conv2/1
  Conv1/1 -> LAS_2AD_mux/1
  or1/1 -> Conv1/1
  CRC/8(output8) -> or8/6
  CRC/7(output7) -> or7/6
  CRC/6(output6) -> or6/6
  CRC/5(output5) -> or5/6
  CRC/4(output4) -> or4/6
  CRC/3(output3) -> or3/6
  CRC/2(output2) -> or2/6
  CRC/1(output1) -> or1/6
  RollingConter/8(output8) -> or8/5
  RollingConter/7(output7) -> or7/5
  RollingConter/6(output6) -> or6/5
  RollingConter/5(output5) -> or5/5
  RollingConter/4(output4) -> or4/5
  RollingConter/3(output3) -> or3/5
  RollingConter/2(output2) -> or2/5
  RollingConter/1(output1) -> or1/5
  LAS_IACCTextInfoForDriver/8(output8) -> or8/4
  LAS_IACCTextInfoForDriver/7(output7) -> or7/4
  LAS_IACCTextInfoForDriver/6(output6) -> or6/4
  LAS_IACCTextInfoForDriver/5(output5) -> or5/4
  LAS_IACCTextInfoForDriver/4(output4) -> or4/4
  LAS_IACCTextInfoForDriver/3(output3) -> or3/4
  LAS_IACCTextInfoForDriver/2(output2) -> or2/4
  LAS_IACCTextInfoForDriver/1(output1) -> or1/4
  LAS_IACCMode/8(output8) -> or8/3
  LAS_IACCMode/7(output7) -> or7/3
  LAS_IACCMode/6(output6) -> or6/3
  LAS_IACCMode/5(output5) -> or5/3
  LAS_IACCMode/4(output4) -> or4/3
  LAS_IACCMode/3(output3) -> or3/3
  LAS_IACCMode/2(output2) -> or2/3
  LAS_IACCMode/1(output1) -> or1/3
  LAS_DriverHandsOff/8(output8) -> or8/2
  LAS_DriverHandsOff/7(output7) -> or7/2
  LAS_DriverHandsOff/6(output6) -> or6/2
  LAS_DriverHandsOff/5(output5) -> or5/2
  LAS_DriverHandsOff/4(output4) -> or4/2
  LAS_DriverHandsOff/3(output3) -> or3/2
  LAS_DriverHandsOff/2(output2) -> or2/2
  LAS_DriverHandsOff/1(output1) -> or1/2
  LAS_TargetBasedLateralCOntrol/8(output8) -> or8/1
  LAS_TargetBasedLateralCOntrol/7(output7) -> or7/1
  LAS_TargetBasedLateralCOntrol/6(output6) -> or6/1
  LAS_TargetBasedLateralCOntrol/5(output5) -> or5/1
  LAS_TargetBasedLateralCOntrol/4(output4) -> or4/1
  LAS_TargetBasedLateralCOntrol/3(output3) -> or3/1
  LAS_TargetBasedLateralCOntrol/2(output2) -> or2/1
  LAS_TargetBasedLateralCOntrol/1(output1) -> or1/1
  LAS_2AD_mux/1 -> output/1

== system VCU_CS75_12_27_test/长安CS75底盘程序，20ms一次/Output/Subsystem/TransmitMessages2/ACC_3C5 ==
  ACC_TargetRange_in : Inport
  ACC_TargetType_in : Inport  Port=2
  RollingConter_in : Inport  Port=3
  CRC_in : Inport  Port=4
  ACC_3C5_DLC : Constant  Value=8  OutDataTypeStr=uint8
  ACC_3C5_DLC_Out : Terminator
  ACC_3C5_ID : Constant  Value=965  OutDataTypeStr=single
  ACC_3C5_ID_Out : Terminator
  ACC_3C5_mux : Mux  Inputs=8
  ACC_TargetRange : Subsystem
  ACC_TargetType : Subsystem
  CRC : Subsystem
  Conv{1..8} (8 alike) : DataTypeConversion
  RollingConter : Subsystem
  or{1..8} (8 alike) : simulink/Logic and Bit Operations/Bitwise Operator  logicop=OR  UseBitMask=off  NumInputPorts=4  BitMask=bin2dec('11011001')  BitMaskRealWorld=Stored Integer
  output : Outport
  wires:
  ACC_3C5_mux/1 -> output/1
  ACC_TargetRange/1(output1) -> or1/1
  ACC_TargetRange/2(output2) -> or2/1
  ACC_TargetRange/3(output3) -> or3/1
  ACC_TargetRange/4(output4) -> or4/1
  ACC_TargetRange/5(output5) -> or5/1
  ACC_TargetRange/6(output6) -> or6/1
  ACC_TargetRange/7(output7) -> or7/1
  ACC_TargetRange/8(output8) -> or8/1
  ACC_TargetType/1(output1) -> or1/2
  ACC_TargetType/2(output2) -> or2/2
  ACC_TargetType/3(output3) -> or3/2
  ACC_TargetType/4(output4) -> or4/2
  ACC_TargetType/5(output5) -> or5/2
  ACC_TargetType/6(output6) -> or6/2
  ACC_TargetType/7(output7) -> or7/2
  ACC_TargetType/8(output8) -> or8/2
  RollingConter/1(output1) -> or1/3
  RollingConter/2(output2) -> or2/3
  RollingConter/3(output3) -> or3/3
  RollingConter/4(output4) -> or4/3
  RollingConter/5(output5) -> or5/3
  RollingConter/6(output6) -> or6/3
  RollingConter/7(output7) -> or7/3
  RollingConter/8(output8) -> or8/3
  CRC/1(output1) -> or1/4
  CRC/2(output2) -> or2/4
  CRC/3(output3) -> or3/4
  CRC/4(output4) -> or4/4
  CRC/5(output5) -> or5/4
  CRC/6(output6) -> or6/4
  CRC/7(output7) -> or7/4
  CRC/8(output8) -> or8/4
  or1/1 -> Conv1/1
  Conv1/1 -> ACC_3C5_mux/1
  or2/1 -> Conv2/1
  Conv2/1 -> ACC_3C5_mux/2
  or3/1 -> Conv3/1
  Conv3/1 -> ACC_3C5_mux/3
  or4/1 -> Conv4/1
  Conv4/1 -> ACC_3C5_mux/4
  or5/1 -> Conv5/1
  Conv5/1 -> ACC_3C5_mux/5
  or6/1 -> Conv6/1
  Conv6/1 -> ACC_3C5_mux/6
  or7/1 -> Conv7/1
  Conv7/1 -> ACC_3C5_mux/7
  or8/1 -> Conv8/1
  Conv8/1 -> ACC_3C5_mux/8
  ACC_3C5_ID/1 -> ACC_3C5_ID_Out/1
  ACC_3C5_DLC/1 -> ACC_3C5_DLC_Out/1
  ACC_TargetRange_in/1 -> ACC_TargetRange/1(ACC_TargetRange)
  ACC_TargetType_in/1 -> ACC_TargetType/1(ACC_TargetType)
  RollingConter_in/1 -> RollingConter/1(RollingConter)
  CRC_in/1 -> CRC/1(CRC)

== system VCU_CS75_12_27_test/长安CS75底盘程序，20ms一次/Output/Subsystem/TransmitMessages3/ACC_3D5 ==
  ACC_LeftTargetLngRange_in : Inport
  ACC_RightTargetDection_in : Inport  Port=2
  ACC_LeftTargetDection_in : Inport  Port=3
  ACC_LeftTargetType_in : Inport  Port=4
  ACC_LeftTargetLatRange_in : Inport  Port=5
  ACC_RightTargetType_in : Inport  Port=6
  ACC_RightTargetLatRange_in : Inport  Port=7
  ACC_RightTargetLngRange_in : Inport  Port=8
  RollingConter_in : Inport  Port=9
  CRC_in : Inport  Port=10
  ACC_3D5_DLC : Constant  Value=8  OutDataTypeStr=uint8
  ACC_3D5_DLC_Out : Terminator
  ACC_3D5_ID : Constant  Value=981  OutDataTypeStr=single
  ACC_3D5_ID_Out : Terminator
  ACC_3D5_mux : Mux  Inputs=8
  ACC_LeftTargetDection : Subsystem
  ACC_LeftTargetLatRange : Subsystem
  ACC_LeftTargetLngRange : Subsystem
  ACC_LeftTargetType : Subsystem
  ACC_RightTargetDection : Subsystem
  ACC_RightTargetLatRange : Subsystem
  ACC_RightTargetLngRange : Subsystem
  ACC_RightTargetType : Subsystem
  CRC : Subsystem
  Conv{1..8} (8 alike) : DataTypeConversion
  RollingConter : Subsystem
  or{1..8} (8 alike) : simulink/Logic and Bit Operations/Bitwise Operator  logicop=OR  UseBitMask=off  NumInputPorts=10  BitMask=bin2dec('11011001')  BitMaskRealWorld=Stored Integer
  output : Outport
  wires:
  ACC_3D5_mux/1 -> output/1
  ACC_LeftTargetLngRange/1(output1) -> or1/1
  ACC_LeftTargetLngRange/2(output2) -> or2/1
  ACC_LeftTargetLngRange/3(output3) -> or3/1
  ACC_LeftTargetLngRange/4(output4) -> or4/1
  ACC_LeftTargetLngRange/5(output5) -> or5/1
  ACC_LeftTargetLngRange/6(output6) -> or6/1
  ACC_LeftTargetLngRange/7(output7) -> or7/1
  ACC_LeftTargetLngRange/8(output8) -> or8/1
  ACC_RightTargetDection/1(output1) -> or1/2
  ACC_RightTargetDection/2(output2) -> or2/2
  ACC_RightTargetDection/3(output3) -> or3/2
  ACC_RightTargetDection/4(output4) -> or4/2
  ACC_RightTargetDection/5(output5) -> or5/2
  ACC_RightTargetDection/6(output6) -> or6/2
  ACC_RightTargetDection/7(output7) -> or7/2
  ACC_RightTargetDection/8(output8) -> or8/2
  ACC_LeftTargetDection/1(output1) -> or1/3
  ACC_LeftTargetDection/2(output2) -> or2/3
  ACC_LeftTargetDection/3(output3) -> or3/3
  ACC_LeftTargetDection/4(output4) -> or4/3
  ACC_LeftTargetDection/5(output5) -> or5/3
  ACC_LeftTargetDection/6(output6) -> or6/3
  ACC_LeftTargetDection/7(output7) -> or7/3
  ACC_LeftTargetDection/8(output8) -> or8/3
  ACC_LeftTargetType/1(output1) -> or1/4
  ACC_LeftTargetType/2(output2) -> or2/4
  ACC_LeftTargetType/3(output3) -> or3/4
  ACC_LeftTargetType/4(output4) -> or4/4
  ACC_LeftTargetType/5(output5) -> or5/4
  ACC_LeftTargetType/6(output6) -> or6/4
  ACC_LeftTargetType/7(output7) -> or7/4
  ACC_LeftTargetType/8(output8) -> or8/4
  ACC_LeftTargetLatRange/1(output1) -> or1/5
  ACC_LeftTargetLatRange/2(output2) -> or2/5
  ACC_LeftTargetLatRange/3(output3) -> or3/5
  ACC_LeftTargetLatRange/4(output4) -> or4/5
  ACC_LeftTargetLatRange/5(output5) -> or5/5
  ACC_LeftTargetLatRange/6(output6) -> or6/5
  ACC_LeftTargetLatRange/7(output7) -> or7/5
  ACC_LeftTargetLatRange/8(output8) -> or8/5
  ACC_RightTargetType/1(output1) -> or1/6
  ACC_RightTargetType/2(output2) -> or2/6
  ACC_RightTargetType/3(output3) -> or3/6
  ACC_RightTargetType/4(output4) -> or4/6
  ACC_RightTargetType/5(output5) -> or5/6
  ACC_RightTargetType/6(output6) -> or6/6
  ACC_RightTargetType/7(output7) -> or7/6
  ACC_RightTargetType/8(output8) -> or8/6
  ACC_RightTargetLatRange/1(output1) -> or1/7
  ACC_RightTargetLatRange/2(output2) -> or2/7
  ACC_RightTargetLatRange/3(output3) -> or3/7
  ACC_RightTargetLatRange/4(output4) -> or4/7
  ACC_RightTargetLatRange/5(output5) -> or5/7
  ACC_RightTargetLatRange/6(output6) -> or6/7
  ACC_RightTargetLatRange/7(output7) -> or7/7
  ACC_RightTargetLatRange/8(output8) -> or8/7
  ACC_RightTargetLngRange/1(output1) -> or1/8
  ACC_RightTargetLngRange/2(output2) -> or2/8
  ACC_RightTargetLngRange/3(output3) -> or3/8
  ACC_RightTargetLngRange/4(output4) -> or4/8
  ACC_RightTargetLngRange/5(output5) -> or5/8
  ACC_RightTargetLngRange/6(output6) -> or6/8
  ACC_RightTargetLngRange/7(output7) -> or7/8
  ACC_RightTargetLngRange/8(output8) -> or8/8
  RollingConter/1(output1) -> or1/9
  RollingConter/2(output2) -> or2/9
  RollingConter/3(output3) -> or3/9
  RollingConter/4(output4) -> or4/9
  RollingConter/5(output5) -> or5/9
  RollingConter/6(output6) -> or6/9
  RollingConter/7(output7) -> or7/9
  RollingConter/8(output8) -> or8/9
  CRC/1(output1) -> or1/10
  CRC/2(output2) -> or2/10
  CRC/3(output3) -> or3/10
  CRC/4(output4) -> or4/10
  CRC/5(output5) -> or5/10
  CRC/6(output6) -> or6/10
  CRC/7(output7) -> or7/10
  CRC/8(output8) -> or8/10
  or1/1 -> Conv1/1
  Conv1/1 -> ACC_3D5_mux/1
  or2/1 -> Conv2/1
  Conv2/1 -> ACC_3D5_mux/2
  or3/1 -> Conv3/1
  Conv3/1 -> ACC_3D5_mux/3
  or4/1 -> Conv4/1
  Conv4/1 -> ACC_3D5_mux/4
  or5/1 -> Conv5/1
  Conv5/1 -> ACC_3D5_mux/5
  or6/1 -> Conv6/1
  Conv6/1 -> ACC_3D5_mux/6
  or7/1 -> Conv7/1
  Conv7/1 -> ACC_3D5_mux/7
  or8/1 -> Conv8/1
  Conv8/1 -> ACC_3D5_mux/8
  ACC_3D5_ID/1 -> ACC_3D5_ID_Out/1
  ACC_3D5_DLC/1 -> ACC_3D5_DLC_Out/1
  ACC_LeftTargetLngRange_in/1 -> ACC_LeftTargetLngRange/1(ACC_LeftTargetLngRange)
  ACC_RightTargetDection_in/1 -> ACC_RightTargetDection/1(ACC_RightTargetDection)
  ACC_LeftTargetDection_in/1 -> ACC_LeftTargetDection/1(ACC_LeftTargetDection)
  ACC_LeftTargetType_in/1 -> ACC_LeftTargetType/1(ACC_LeftTargetType)
  ACC_LeftTargetLatRange_in/1 -> ACC_LeftTargetLatRange/1(ACC_LeftTargetLatRange)
  ACC_RightTargetType_in/1 -> ACC_RightTargetType/1(ACC_RightTargetType)
  ACC_RightTargetLatRange_in/1 -> ACC_RightTargetLatRange/1(ACC_RightTargetLatRange)
  ACC_RightTargetLngRange_in/1 -> ACC_RightTargetLngRange/1(ACC_RightTargetLngRange)
  RollingConter_in/1 -> RollingConter/1(RollingConter)
  CRC_in/1 -> CRC/1(CRC)

== system VCU_CS75_12_27_test/长安CS75底盘程序，20ms一次/Output/Subsystem/TransmitMessages4/ACC_3E5 ==
  ACC_SetSpeedDisplay_in : Inport
  ACC_ObjValid_in : Inport  Port=2
  ACC_TimeGapSet_in : Inport  Port=3
  ACC_DistanceTarObj_in : Inport  Port=4
  ACC_ControlType_in : Inport  Port=5
  ACC_takeoverRequesr_in : Inport  Port=6
  ACC_ACCObjEnableStatus_in : Inport  Port=7
  ACC_FCWSensityStatus_in : Inport  Port=8
  ACC_FCWEnableStatus_in : Inport  Port=9
  RollingConter_in : Inport  Port=10
  ACC_EPBReq_in : Inport  Port=11
  ACC_AutoBrakeEnableStatus_in : Inport  Port=12
  CRC_in : Inport  Port=13
  ACC_3E5_DLC : Constant  Value=8  OutDataTypeStr=uint8
  ACC_3E5_DLC_Out : Terminator
  ACC_3E5_ID : Constant  Value=997  OutDataTypeStr=single
  ACC_3E5_ID_Out : Terminator
  ACC_3E5_mux : Mux  Inputs=8
  ACC_ACCObjEnableStatus : Subsystem
  ACC_AutoBrakeEnableStatus : Subsystem
  ACC_ControlType : Subsystem
  ACC_DistanceTarObj : Subsystem
  ACC_EPBReq : Subsystem
  ACC_FCWEnableStatus : Subsystem
  ACC_FCWSensityStatus : Subsystem
  ACC_ObjValid : Subsystem
  ACC_SetSpeedDisplay : Subsystem
  ACC_TimeGapSet : Subsystem
  ACC_takeoverRequesr : Subsystem
  CRC : Subsystem
  Conv{1..8} (8 alike) : DataTypeConversion
  RollingConter : Subsystem
  or{1..8} (8 alike) : simulink/Logic and Bit Operations/Bitwise Operator  logicop=OR  UseBitMask=off  NumInputPorts=13  BitMask=bin2dec('11011001')  BitMaskRealWorld=Stored Integer
  output : Outport
  wires:
  CRC_in/1 -> CRC/1(CRC)
  ACC_AutoBrakeEnableStatus_in/1 -> ACC_AutoBrakeEnableStatus/1(ACC_AutoBrakeEnableStatus)
  ACC_EPBReq_in/1 -> ACC_EPBReq/1(ACC_EPBReq)
  RollingConter_in/1 -> RollingConter/1(RollingConter)
  ACC_FCWEnableStatus_in/1 -> ACC_FCWEnableStatus/1(ACC_FCWEnableStatus)
  ACC_FCWSensityStatus_in/1 -> ACC_FCWSensityStatus/1(ACC_FCWSensityStatus)
  ACC_ACCObjEnableStatus_in/1 -> ACC_ACCObjEnableStatus/1(ACC_ACCObjEnableStatus)
  ACC_takeoverRequesr_in/1 -> ACC_takeoverRequesr/1(ACC_takeoverRequesr)
  ACC_ControlType_in/1 -> ACC_ControlType/1(ACC_ControlType)
  ACC_DistanceTarObj_in/1 -> ACC_DistanceTarObj/1(ACC_DistanceTarObj)
  ACC_TimeGapSet_in/1 -> ACC_TimeGapSet/1(ACC_TimeGapSet)
  ACC_ObjValid_in/1 -> ACC_ObjValid/1(ACC_ObjValid)
  ACC_SetSpeedDisplay_in/1 -> ACC_SetSpeedDisplay/1(ACC_SetSpeedDisplay)
  ACC_3E5_DLC/1 -> ACC_3E5_DLC_Out/1
  ACC_3E5_ID/1 -> ACC_3E5_ID_Out/1
  Conv8/1 -> ACC_3E5_mux/8
  or8/1 -> Conv8/1
  Conv7/1 -> ACC_3E5_mux/7
  or7/1 -> Conv7/1
  Conv6/1 -> ACC_3E5_mux/6
  or6/1 -> Conv6/1
  Conv5/1 -> ACC_3E5_mux/5
  or5/1 -> Conv5/1
  Conv4/1 -> ACC_3E5_mux/4
  or4/1 -> Conv4/1
  Conv3/1 -> ACC_3E5_mux/3
  or3/1 -> Conv3/1
  Conv2/1 -> ACC_3E5_mux/2
  or2/1 -> Conv2/1
  Conv1/1 -> ACC_3E5_mux/1
  or1/1 -> Conv1/1
  CRC/8(output8) -> or8/13
  CRC/7(output7) -> or7/13
  CRC/6(output6) -> or6/13
  CRC/5(output5) -> or5/13
  CRC/4(output4) -> or4/13
  CRC/3(output3) -> or3/13
  CRC/2(output2) -> or2/13
  CRC/1(output1) -> or1/13
  ACC_AutoBrakeEnableStatus/8(output8) -> or8/12
  ACC_AutoBrakeEnableStatus/7(output7) -> or7/12
  ACC_AutoBrakeEnableStatus/6(output6) -> or6/12
  ACC_AutoBrakeEnableStatus/5(output5) -> or5/12
  ACC_AutoBrakeEnableStatus/4(output4) -> or4/12
  ACC_AutoBrakeEnableStatus/3(output3) -> or3/12
  ACC_AutoBrakeEnableStatus/2(output2) -> or2/12
  ACC_AutoBrakeEnableStatus/1(output1) -> or1/12
  ACC_EPBReq/8(output8) -> or8/11
  ACC_EPBReq/7(output7) -> or7/11
  ACC_EPBReq/6(output6) -> or6/11
  ACC_EPBReq/5(output5) -> or5/11
  ACC_EPBReq/4(output4) -> or4/11
  ACC_EPBReq/3(output3) -> or3/11
  ACC_EPBReq/2(output2) -> or2/11
  ACC_EPBReq/1(output1) -> or1/11
  RollingConter/8(output8) -> or8/10
  RollingConter/7(output7) -> or7/10
  RollingConter/6(output6) -> or6/10
  RollingConter/5(output5) -> or5/10
  RollingConter/4(output4) -> or4/10
  RollingConter/3(output3) -> or3/10
  RollingConter/2(output2) -> or2/10
  RollingConter/1(output1) -> or1/10
  ACC_FCWEnableStatus/8(output8) -> or8/9
  ACC_FCWEnableStatus/7(output7) -> or7/9
  ACC_FCWEnableStatus/6(output6) -> or6/9
  ACC_FCWEnableStatus/5(output5) -> or5/9
  ACC_FCWEnableStatus/4(output4) -> or4/9
  ACC_FCWEnableStatus/3(output3) -> or3/9
  ACC_FCWEnableStatus/2(output2) -> or2/9
  ACC_FCWEnableStatus/1(output1) -> or1/9
  ACC_FCWSensityStatus/8(output8) -> or8/8
  ACC_FCWSensityStatus/7(output7) -> or7/8
  ACC_FCWSensityStatus/6(output6) -> or6/8
  ACC_FCWSensityStatus/5(output5) -> or5/8
  ACC_FCWSensityStatus/4(output4) -> or4/8
  ACC_FCWSensityStatus/3(output3) -> or3/8
  ACC_FCWSensityStatus/2(output2) -> or2/8
  ACC_FCWSensityStatus/1(output1) -> or1/8
  ACC_ACCObjEnableStatus/8(output8) -> or8/7
  ACC_ACCObjEnableStatus/7(output7) -> or7/7
  ACC_ACCObjEnableStatus/6(output6) -> or6/7
  ACC_ACCObjEnableStatus/5(output5) -> or5/7
  ACC_ACCObjEnableStatus/4(output4) -> or4/7
  ACC_ACCObjEnableStatus/3(output3) -> or3/7
  ACC_ACCObjEnableStatus/2(output2) -> or2/7
  ACC_ACCObjEnableStatus/1(output1) -> or1/7
  ACC_takeoverRequesr/8(output8) -> or8/6
  ACC_takeoverRequesr/7(output7) -> or7/6
  ACC_takeoverRequesr/6(output6) -> or6/6
  ACC_takeoverRequesr/5(output5) -> or5/6
  ACC_takeoverRequesr/4(output4) -> or4/6
  ACC_takeoverRequesr/3(output3) -> or3/6
  ACC_takeoverRequesr/2(output2) -> or2/6
  ACC_takeoverRequesr/1(output1) -> or1/6
  ACC_ControlType/8(output8) -> or8/5
  ACC_ControlType/7(output7) -> or7/5
  ACC_ControlType/6(output6) -> or6/5
  ACC_ControlType/5(output5) -> or5/5
  ACC_ControlType/4(output4) -> or4/5
  ACC_ControlType/3(output3) -> or3/5
  ACC_ControlType/2(output2) -> or2/5
  ACC_ControlType/1(output1) -> or1/5
  ACC_DistanceTarObj/8(output8) -> or8/4
  ACC_DistanceTarObj/7(output7) -> or7/4
  ACC_DistanceTarObj/6(output6) -> or6/4
  ACC_DistanceTarObj/5(output5) -> or5/4
  ACC_DistanceTarObj/4(output4) -> or4/4
  ACC_DistanceTarObj/3(output3) -> or3/4
  ACC_DistanceTarObj/2(output2) -> or2/4
  ACC_DistanceTarObj/1(output1) -> or1/4
  ACC_TimeGapSet/8(output8) -> or8/3
  ACC_TimeGapSet/7(output7) -> or7/3
  ACC_TimeGapSet/6(output6) -> or6/3
  ACC_TimeGapSet/5(output5) -> or5/3
  ACC_TimeGapSet/4(output4) -> or4/3
  ACC_TimeGapSet/3(output3) -> or3/3
  ACC_TimeGapSet/2(output2) -> or2/3
  ACC_TimeGapSet/1(output1) -> or1/3
  ACC_ObjValid/8(output8) -> or8/2
  ACC_ObjValid/7(output7) -> or7/2
  ACC_ObjValid/6(output6) -> or6/2
  ACC_ObjValid/5(output5) -> or5/2
  ACC_ObjValid/4(output4) -> or4/2
  ACC_ObjValid/3(output3) -> or3/2
  ACC_ObjValid/2(output2) -> or2/2
  ACC_ObjValid/1(output1) -> or1/2
  ACC_SetSpeedDisplay/8(output8) -> or8/1
  ACC_SetSpeedDisplay/7(output7) -> or7/1
  ACC_SetSpeedDisplay/6(output6) -> or6/1
  ACC_SetSpeedDisplay/5(output5) -> or5/1
  ACC_SetSpeedDisplay/4(output4) -> or4/1
  ACC_SetSpeedDisplay/3(output3) -> or3/1
  ACC_SetSpeedDisplay/2(output2) -> or2/1
  ACC_SetSpeedDisplay/1(output1) -> or1/1
  ACC_3E5_mux/1 -> output/1
